simulink model "GenerateImageDataOfParkingLot"  (R2021b)
settings: Solver=VariableStepAuto  StartTime=0.0  StopTime=60  RelTol=1e-3
values from neighbouring files (symbols this model uses):
  baseline = 0.5    [DevelopVisualSLAMAlgorithmUsingUnrealEngineSimulationExample.m]
  refPosesT = data.refPosesT    [DevelopVisualSLAMAlgorithmUsingUnrealEngineSimulationExample.m]    (also in parkingLotReferenceData.mat = [0 0.0660467506529 0.132094151907 0.198142181103 0.264190812)
  refPosesX = data.refPosesX    [DevelopVisualSLAMAlgorithmUsingUnrealEngineSimulationExample.m]    (also in parkingLotReferenceData.mat = [0 0.0660467506529 0.132094151907 0.198142181103 0.264190812)
  refPosesY = data.refPosesY    [DevelopVisualSLAMAlgorithmUsingUnrealEngineSimulationExample.m]    (also in parkingLotReferenceData.mat = [0 0.0660467506529 0.132094151907 0.198142181103 0.264190812)
undefined symbols (not defined in the file or in its folder): gray
libraries: sim3dcameralib x3, sim3dlib x1, sim3dautolib x1
settings Model: Creator=The MathWorks, Inc.  LastModifiedBy=The MathWorks, Inc.
settings SolverCC: AlgebraicLoopSolver=TrustRegion
settings DebuggingCC: SymbolicDimsDataTypeCodeGenerationDiagnostic=none  SFMachineParentedDataDiag=warning

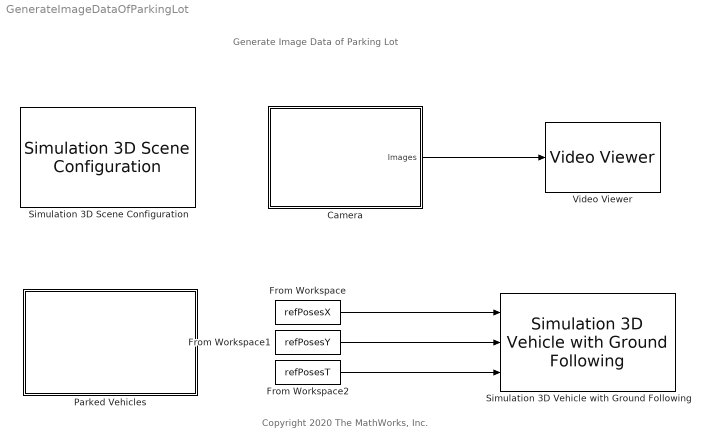
== system GenerateImageDataOfParkingLot ==
  note: Generate Image Data of Parking Lot
  note: Copyright 2020 The MathWorks, Inc.
  Camera : Subsystem  Variant=on
  From Workspace : FromWorkspace  VariableName=refPosesX
  From Workspace1 : FromWorkspace  VariableName=refPosesY
  From Workspace2 : FromWorkspace  VariableName=refPosesT
  Parked Vehicles : Subsystem
  Simulation 3D Scene Configuration : sim3dlib/Simulation 3D Scene Configuration  Priority=0  ProjectFormat_internal=Default Scenes  ProjectFormat=Default Scenes  SceneDesc=Large parking lot  ProjectName=/mathworks/devel/bat/BR2021bd/build/matlab/toolbox/shared/sim3d_projects/automotive_project/UE4/LinuxNoEditor/AutoVrtlEnv.sh  ScenePath=/Game/Maps/HwStrght  vehTagList={'Scene Origin';'SimulinkVehicle1'}  vehTag=SimulinkVehicle1  OpVisEn=off  Ts=0.04  EnableWindow=on  EnableWeather=off  SunAltitude=40.0  SunAzimuth=90  clouds=10  wind=1  fog=0  rain=0  sensorTag=MainCamera2  sensorId=2  sensorName=MainCamera2  mountLoc=Origin  offsetFlag=off  tmountOffset=[0, 0, 0]  rmountOffset=[0, 0, 0]  HorizontalResolution=1280  VerticalResolution=720  HorizontalFOV=60  mountPoint=[0 0 0]  mountOrientation=[0 0 0]  aMode=3  ID=2
      settings: SourceProductBaseCode=AE,DR,UV,VE
  Simulation 3D Vehicle with Ground Following : sim3dautolib/Simulation 3D Vehicle with Ground Following  Priority=-1  PassVehMesh=Hatchback  PassVehMesh_Internal=Muscle car  MeshPath=/MathWorksSimulation/Vehicles/Muscle/Meshes/SK_MuscleCar.SK_MuscleCar  TrackWidth=1.9  WheelBase=3  WheelRadius=0.35  VehColor=Red  VehColor_Internal=Red  InitialPos=[refPosesX(1,2), refPosesY(1,2), 0]  InitialRot=[0, 0, refPosesT(1,2)]  ActorName=SimulinkVehicle1  SampleTime=-1  ActorType=SimulinkVehicle  ID=1  aMode=3  ActorTag=SimulinkVehicle1  CoordinateScheme=ISO  VehLightsControl=off  HeadlightColor=[ 1, 1, 1 ]  HighBeamIntensity=100000  LowBeamIntensity=60000  HighBeamConeAngle=70  LowBeamConeAngle=70  LeftHeadlightOrientation=[ 0, 0 ]  RightHeadlightOrientation=[ 0, 0 ]  BrakelightIntensity=500  ReverselightIntensity=500  SignallightIntensity=500  SignallightPeriod=1  SignalPulseWidth=50  TransformOutportEnabled=off
      settings: SourceProductBaseCode=AE,DR,UV,VE
  Video Viewer : VideoViewer  colormapValue=gray(256)  FigPos=[899 940 1214 789]
  wires:
  From Workspace/1 -> Simulation 3D Vehicle with Ground Following/1
  From Workspace1/1 -> Simulation 3D Vehicle with Ground Following/2
  From Workspace2/1 -> Simulation 3D Vehicle with Ground Following/3
  Camera/1(Images) -> Video Viewer/1

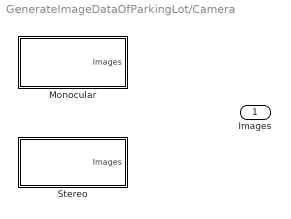
== system GenerateImageDataOfParkingLot/Camera ==
  Monocular : Subsystem  VariantControl=useMonoCamera == 1
  Stereo : Subsystem  VariantControl=useMonoCamera == 0
  Images : Outport

== system GenerateImageDataOfParkingLot/Parked Vehicles ==

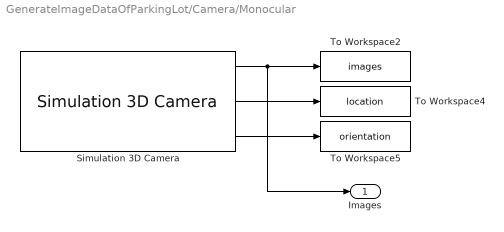
== system GenerateImageDataOfParkingLot/Camera/Monocular ==
  Simulation 3D Camera : sim3dcameralib/Simulation 3D Camera  Priority=1  sensorTag=Sim3dSensor7  sensorId=7  sensorName=Sim3dSensor7  vehTagList={'Scene Origin';'SimulinkVehicle1'}  vehTag=SimulinkVehicle1  mountLoc=Roof center  offsetFlag=off  tmountOffset=[0, 0, 0]  extTmount=off  rmountOffset=[0, 0, 0]  extRmount=off  FocalLength=focalLength  OpticalCenter=principalPoint  ImageSize=imageSize  RadialDistortion=[0, 0]  TangentialDistortion=[0, 0]  SensorSkew=0  DepthOutportEnabled=off  SemanticOutportEnabled=off  TransformOutportEnabled=on  SampleTime=-1  mountPoint=[0 0 1.55999994277954]  mountOrientation=[0 0 0]  aMode=3  ID=7
      settings: SourceProductBaseCode=AE,DR,UV,VE
  To Workspace2 : ToWorkspace  VariableName=images  SaveFormat=Timeseries  SampleTime=-1
  To Workspace4 : ToWorkspace  VariableName=location  SaveFormat=Timeseries  SampleTime=-1
  To Workspace5 : ToWorkspace  VariableName=orientation  SaveFormat=Timeseries  SampleTime=-1
  Images : Outport
  wires:
  Simulation 3D Camera/2 -> To Workspace4/1
  Simulation 3D Camera/3 -> To Workspace5/1
  Simulation 3D Camera/1 -> Images/1, To Workspace2/1

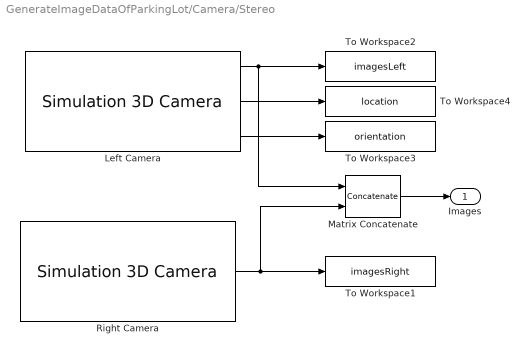
== system GenerateImageDataOfParkingLot/Camera/Stereo ==
  Left Camera : sim3dcameralib/Simulation 3D Camera  Priority=1  sensorTag=Sim3dSensor5  sensorId=5  sensorName=Sim3dSensor5  vehTagList={'Scene Origin';'SimulinkVehicle1'}  vehTag=SimulinkVehicle1  mountLoc=Roof center  offsetFlag=on  tmountOffset=[0, baseline/2, 0]  extTmount=off  rmountOffset=[0, 0, 0]  extRmount=off  FocalLength=focalLength  OpticalCenter=principalPoint  ImageSize=imageSize  RadialDistortion=[0, 0]  TangentialDistortion=[0, 0]  SensorSkew=0  DepthOutportEnabled=off  SemanticOutportEnabled=off  TransformOutportEnabled=on  SampleTime=-1  mountPoint=[0 -0.25 1.55999994277954]  mountOrientation=[0 0 0]  aMode=3  ID=5
      settings: SourceProductBaseCode=AE,DR,UV,VE
  Matrix Concatenate : Concatenate  Mode=Multidimensional array
  Right Camera : sim3dcameralib/Simulation 3D Camera  Priority=1  sensorTag=Sim3dSensor6  sensorId=6  sensorName=Sim3dSensor6  vehTagList={'Scene Origin';'SimulinkVehicle1'}  vehTag=SimulinkVehicle1  mountLoc=Roof center  offsetFlag=on  tmountOffset=[0, -baseline/2, 0]  extTmount=off  rmountOffset=[0, 0, 0]  extRmount=off  FocalLength=focalLength  OpticalCenter=principalPoint  ImageSize=imageSize  RadialDistortion=[0, 0]  TangentialDistortion=[0, 0]  SensorSkew=0  DepthOutportEnabled=off  SemanticOutportEnabled=off  TransformOutportEnabled=off  SampleTime=-1  mountPoint=[0 0.25 1.55999994277954]  mountOrientation=[0 0 0]  aMode=3  ID=6
      settings: SourceProductBaseCode=AE,DR,UV,VE
  To Workspace1 : ToWorkspace  VariableName=imagesRight  SaveFormat=Timeseries  SampleTime=-1
  To Workspace2 : ToWorkspace  VariableName=imagesLeft  SaveFormat=Timeseries  SampleTime=-1
  To Workspace3 : ToWorkspace  VariableName=orientation  SaveFormat=Timeseries  SampleTime=-1
  To Workspace4 : ToWorkspace  VariableName=location  SaveFormat=Timeseries  SampleTime=-1
  Images : Outport
  wires:
  Matrix Concatenate/1 -> Images/1
  Left Camera/2 -> To Workspace4/1
  Left Camera/1 -> To Workspace2/1, Matrix Concatenate/1
  Left Camera/3 -> To Workspace3/1
  Right Camera/1 -> To Workspace1/1, Matrix Concatenate/2
